simulink model "nomoto_2_order"  (R2017b)
settings: Solver=VariableStepAuto  StartTime=0.0  StopTime=30000  RelTol=1e-3
values from neighbouring files (symbols this model uses):
  b = 0.001    [task_2_4.m]
  K = 0.1    [task_2_4.m]
  k_d = 1e-2    (= 0.01)    [task_2_4.m]
  k_i = 0e-8    (= 0)    [task_2_4.m]
  k_p = 5e-5    (= 5e-05)    [task_2_4.m]
  T = 20    [task_2_4.m]
  U = 5    [task_2_4.m]
libraries: simulink x1
settings Model: Creator=Ivan  LastModifiedBy=Ivan

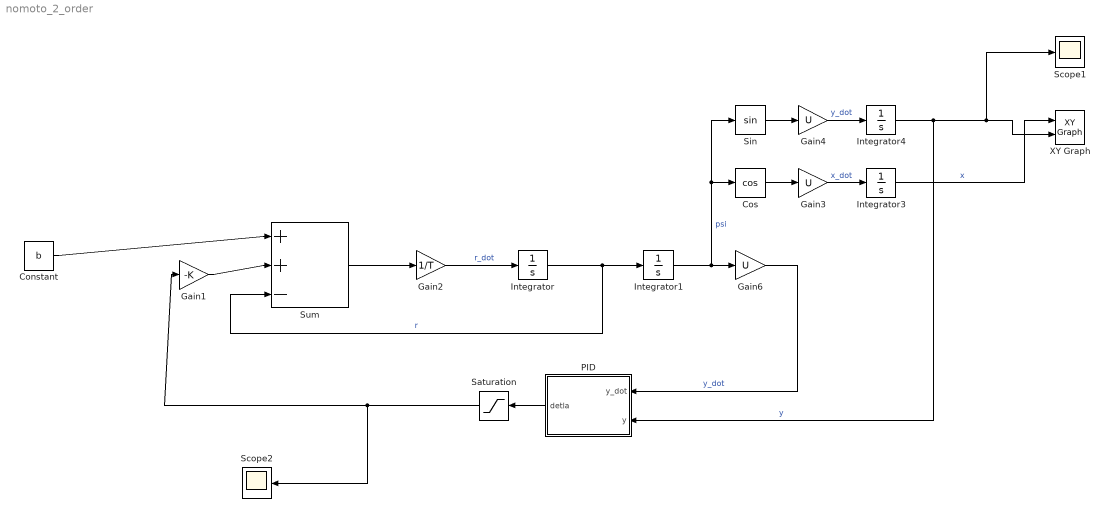
== system nomoto_2_order ==
  Constant : Constant  Value=b
  Cos : Trigonometry  Operator=cos
  Gain1 : Gain  Gain=-K
  Gain2 : Gain  Gain=1/T
  Gain3 : Gain  Gain=U
  Gain4 : Gain  Gain=U
  Gain6 : Gain  Gain=U
  Integrator : Integrator
  Integrator1 : Integrator
  Integrator3 : Integrator
  Integrator4 : Integrator  InitialCondition=100
  PID : Subsystem
  Saturation : Saturate  UpperLimit=0.35  LowerLimit=-0.35
  Scope1 : Scope
  Scope2 : Scope
  Sin : Trigonometry
  Sum : Sum  Inputs=|++-
  XY Graph : simulink/Sinks/XY Graph  xmin=0  xmax=100000  ymin=-500  ymax=500  st=-1
  wires:
  Sum/1 -> Gain2/1
  Constant/1 -> Sum/1
  Gain2/1 -> Integrator/1  "r_dot"
  Integrator/1 -> Sum/3, Integrator1/1  "r"
  Gain1/1 -> Sum/2
  Integrator1/1 -> Gain6/1, Sin/1, Cos/1  "psi"
  Gain6/1 -> PID/1(y_dot)  "y_dot"
  PID/1(detla) -> Saturation/1
  Cos/1 -> Gain3/1
  Gain3/1 -> Integrator3/1  "x_dot"
  Gain4/1 -> Integrator4/1  "y_dot"
  Sin/1 -> Gain4/1
  Integrator4/1 -> PID/2(y), Scope1/1, XY Graph/2  "y"
  Integrator3/1 -> XY Graph/1  "x"
  Saturation/1 -> Scope2/1, Gain1/1

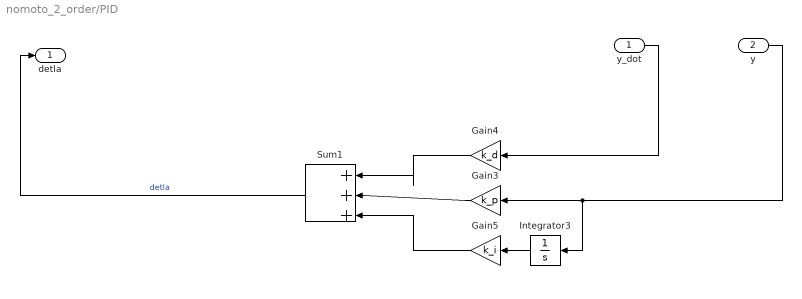
== system nomoto_2_order/PID ==
  y_dot : Inport
  y : Inport  Port=2
  Gain3 : Gain  Gain=k_p
  Gain4 : Gain  Gain=k_d
  Gain5 : Gain  Gain=k_i
  Integrator3 : Integrator
  Sum1 : Sum  Inputs=|+++
  detla : Outport
  wires:
  y_dot/1 -> Gain4/1
  y/1 -> Integrator3/1, Gain3/1
  Gain5/1 -> Sum1/3
  Sum1/1 -> detla/1  "detla"
  Integrator3/1 -> Gain5/1
  Gain4/1 -> Sum1/1
  Gain3/1 -> Sum1/2
